simulink model "MRAS"  (R2018a)
settings: Solver=VariableStepAuto  StartTime=0.0  StopTime=100  RelTol=1e-3
settings Model: Creator=edward  LastModifiedBy=edward

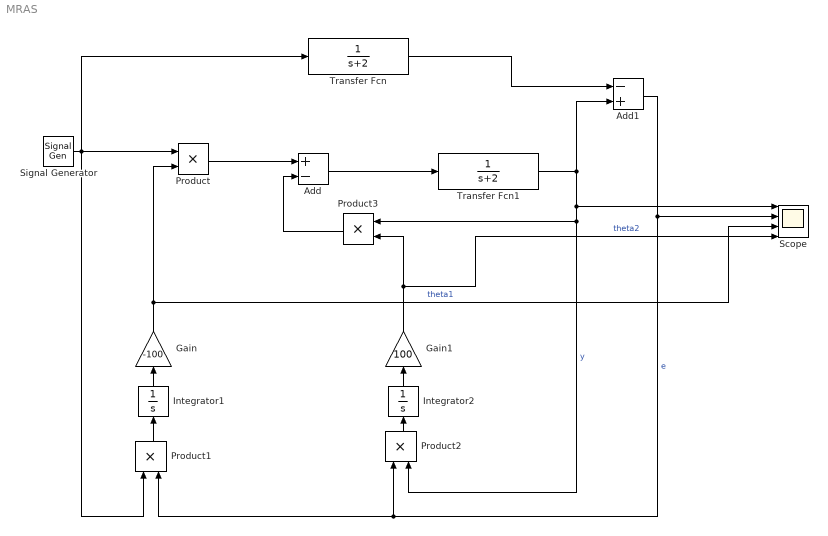
== system MRAS ==
  Add : Sum  Inputs=+-
  Add1 : Sum  Inputs=-+
  Gain : Gain  Gain=-100
  Gain1 : Gain  Gain=100
  Integrator1 : Integrator
  Integrator2 : Integrator
  Product{,1..3} (4 alike) : Product
  Scope : Scope  NumInputPorts=4
  Signal Generator : SignalGenerator  WaveForm=square  Frequency=0.5  Units=rad/sec
  Transfer Fcn : TransferFcn  Denominator=[1 2]
  Transfer Fcn1 : TransferFcn  Denominator=[1 2]
  wires:
  Product1/1 -> Integrator1/1
  Product2/1 -> Integrator2/1
  Add1/1 -> Product2/1, Product1/2, Scope/2  "e"
  Signal Generator/1 -> Transfer Fcn/1, Product1/1, Product/1
  Transfer Fcn/1 -> Add1/1
  Transfer Fcn1/1 -> Scope/1, Product3/1, Product2/2, Add1/2  "y"
  Integrator2/1 -> Gain1/1
  Product3/1 -> Add/2
  Product/1 -> Add/1
  Add/1 -> Transfer Fcn1/1
  Integrator1/1 -> Gain/1
  Gain1/1 -> Product3/2, Scope/4  "theta2"
  Gain/1 -> Scope/3, Product/2  "theta1"
